simulink model "Q_2"  (R2019a)
settings: Solver=ode4  StartTime=0.0  StopTime=80  FixedStep=0.001  RelTol=1e-3  EnableMultiTasking=on
undefined symbols (not defined in the file or in its folder): attitude_control_1
settings Model: Creator=dell-  LastModifiedBy=lx
settings DataIOCC: LimitDataPoints=on  SaveFormat=Array  ReturnWorkspaceOutputs=off
settings OptimizationCC: LifeSpan=inf
settings DebuggingCC: SolverPrmCheckMsg=warning  SFUnexpectedBacktrackingDiag=warning  SFNoUnconditionalDefaultTransitionDiag=warning  SFExecutionAtInitializationDiag=none  ArithmeticOperatorsInVariantConditions=warning
settings HardwareCC: ProdBitPerPointer=32  ProdBitPerSizeT=32  ProdBitPerPtrDiffT=32  ProdLargestAtomicFloat=None  ProdIntDivRoundTo=Undefined  ProdEndianess=Unspecified  ProdWordSize=32  ProdHWDeviceType=32-bit Generic
settings ModelReferenceCC: PropagateSignalLabelsOutOfModel=off
settings SFSimCC: SimUseLocalCustomCode=off
settings RTWCC: RTWUseLocalCustomCode=off
settings CodeAppCC: StateflowObjectComments=on
settings GRTTargetCC: TargetLangStandard=C89/C90 (ANSI)  GeneratePreprocessorConditionals=Disable all
settings ConfigComp: CovMetricSettings=dw  CovHtmlReporting=on  CovSaveCumulativeToWorkspaceVar=on  CovSaveSingleToWorkspaceVar=on  CovExternalEMLEnable=off  CovSFcnEnable=off

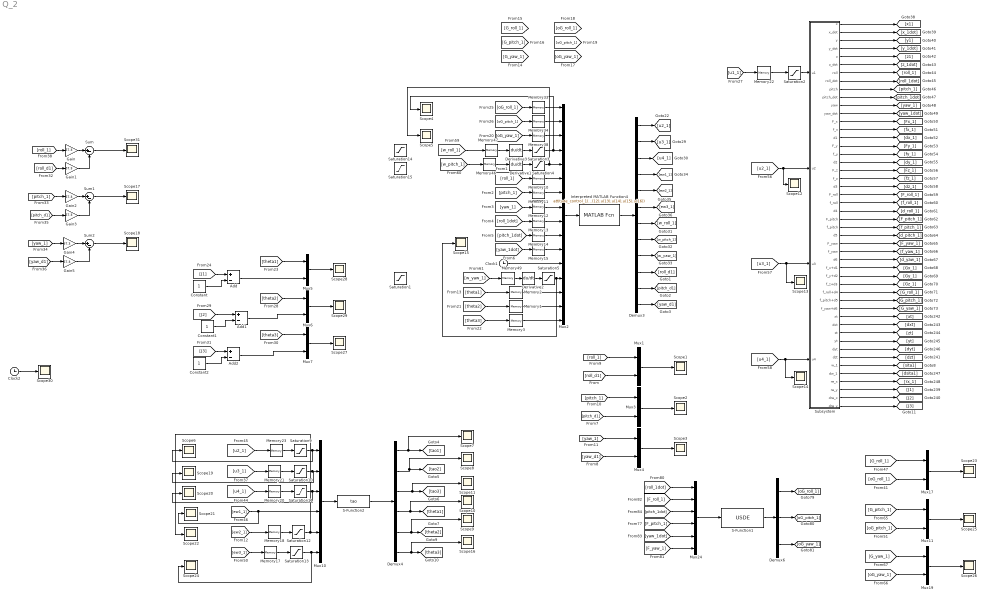
== system Q_2 ==
  Add : Sum  Inputs=+-
  Add1 : Sum  Inputs=+-
  Add2 : Sum  Inputs=+-
  Clock1 : Clock
  Clock2 : Clock
  Constant : Constant
  Constant1 : Constant
  Constant2 : Constant
  Demux3 : Demux  Outputs=12
  Demux4 : Demux  Outputs=6
  Demux6 : Demux  Outputs=3
  Derivative1 : Derivative
  Derivative2 : Derivative
  Derivative3 : Derivative
  Gain{,1..5} (6 alike) : Gain  Gain=57.3
  Interpreted MATLAB Function4 : MATLABFcn  MATLABFcn=attitude_control_1(u(1),u(2),u(3),u(4),u(5),u(6),u(7),u(8),u(9),u(10),u(11),u(12),u(13),u(14),u(15),u(16))  OutputDimensions=12  SampleTime=0.001
  Memory1 : Memory  InitialCondition=5.5
  Memory{10..11,13..15,18,20..23,33..34,38,46..47,49} (16 alike) : Memory
  Memory12 : Memory  InitialCondition=0.2
  Memory17 : Memory  InitialCondition=1
  Memory2 : Memory  InitialCondition=6
  Memory3 : Memory  InitialCondition=3
  Mux{1,3..7,11,17,19} (9 alike) : Mux  Inputs=2
  Mux10 : Mux  Inputs=6
  Mux2 : Mux  Inputs=16
  Mux24 : Mux  Inputs=6
  S-Function1 : S-Function  Priority=2  FunctionName=USDE  SFunctionDeploymentMode=off  EnableBusSupport=off
  S-Function2 : S-Function  FunctionName=tao  SFunctionDeploymentMode=off  EnableBusSupport=off
  Saturation1 : Saturate  UpperLimit=0.1  LowerLimit=-0.1
  Saturation10 : Saturate  UpperLimit=1.5  LowerLimit=-1
  Saturation11 : Saturate  UpperLimit=5  LowerLimit=-5
  Saturation12 : Saturate
  Saturation13 : Saturate  UpperLimit=0.2  LowerLimit=-0.2
  Saturation14 : Saturate  UpperLimit=0.2  LowerLimit=-0.2
  Saturation15 : Saturate
  Saturation2 : Saturate  UpperLimit=75  LowerLimit=-75
  Saturation3 : Saturate  UpperLimit=0.2  LowerLimit=-0.2
  Saturation4 : Saturate
  Saturation5 : Saturate  UpperLimit=0.1  LowerLimit=-0.1
  Saturation9 : Saturate  UpperLimit=1  LowerLimit=-1
  Scope{1..31} (31 alike) : Scope
  Subsystem : Subsystem  TreatAsAtomicUnit=on
      settings: RTWFcnNameOpts=Use subsystem name  RTWFileNameOpts=Use function name
  Sum : Sum  Inputs=|+-
  Sum1 : Sum  Inputs=|+-
  Sum2 : Sum  Inputs=|+-
  wires:
  [u1_1] -> Memory22/1
  [u2_1] -> Scope12/1, Subsystem/2(u2)
  [u3_1] -> Scope13/1, Subsystem/3(u3)
  [u4_1] -> Scope14/1, Subsystem/4(u4)
  Subsystem/1(x) -> [x1]
  Subsystem/2(x_dot) -> [x_1dot]
  Subsystem/3(y) -> [y1]
  Subsystem/4(y_dot) -> [y_1dot]
  Subsystem/5(z) -> [z1]
  Subsystem/6(z_dot) -> [z_1dot]
  Subsystem/7(roll) -> [roll_1]
  Subsystem/8(roll_dot) -> [roll_1dot]
  Subsystem/9(pitch) -> [pitch_1]
  Subsystem/10(pitch_dot) -> [pitch_1dot]
  Subsystem/11(yaw) -> [yaw_1]
  Subsystem/12(yaw_dot) -> [yaw_1dot]
  Subsystem/13(F_x) -> [Fx_1]
  Subsystem/14(f_x) -> [fx_1]
  Subsystem/15(d1) -> [dx_1]
  Subsystem/16(F_y) -> [Fy_1]
  Subsystem/17(f_y) -> [fy_1]
  Subsystem/18(d2) -> [dy_1]
  Subsystem/19(F_z) -> [Fz_1]
  Subsystem/20(f_z) -> [fz_1]
  Subsystem/21(d3) -> [dz_1]
  Subsystem/22(F_roll) -> [F_roll_1]
  Subsystem/23(f_roll) -> [f_roll_1]
  Subsystem/24(d4) -> [d_roll_1]
  Subsystem/25(F_pitch) -> [F_pitch_1]
  Subsystem/26(f_pitch) -> [f_pitch_1]
  Subsystem/27(d5) -> [d_pitch_1]
  Subsystem/28(F_yaw) -> [F_yaw_1]
  Subsystem/29(f_yaw) -> [f_yaw_1]
  Subsystem/30(d6) -> [d_yaw_1]
  Subsystem/36(f_yaw+d6) -> [G_yaw_1]
  Subsystem/35(f_pitch+d5) -> [G_pitch_1]
  Subsystem/34(f_roll+d4) -> [G_roll_1]
  Subsystem/33(f_z+d3) -> [Gz_1]
  Subsystem/32(f_y+d2) -> [Gy_1]
  Subsystem/31(f_x+d1) -> [Gx_1]
  Subsystem/41(dyt) -> [dyt]
  Subsystem/40(yt) -> [yt]
  Subsystem/39(zt) -> [zt]
  Subsystem/38(dxt) -> [dxt]
  Subsystem/42(dzt) -> [dzt]
  Subsystem/44(dw_1) -> [dsita1]
  Subsystem/45(re_x) -> [rx_1]
  Subsystem/46(re_y) -> [J1]
  Subsystem/47(dre_x) -> [J2]
  Subsystem/48(dre_y) -> [J3]
  Subsystem/37(xt) -> [xt]
  Interpreted MATLAB Function4/1 -> Demux3/1
  Mux2/1 -> Interpreted MATLAB Function4/1
  [oG_pitch_1] -> Memory34/1
  [oG_yaw_1] -> Memory38/1
  [oG_roll_1] -> Memory33/1
  Memory33/1 -> Mux2/1
  Memory34/1 -> Mux2/2
  Memory38/1 -> Mux2/3
  [roll_1] -> Memory10/1
  [yaw_1] -> Memory12/1
  [pitch_1] -> Memory11/1
  [roll_1dot] -> Memory13/1
  [pitch_1dot] -> Memory14/1
  [yaw_1dot] -> Memory15/1
  Demux3/4 -> [ew1_1]
  Demux3/5 -> [ew2_1]
  Demux3/6 -> [ew3_1]
  Demux3/1 -> [u2_1]
  Demux3/2 -> [u3_1]
  Demux3/3 -> [u4_1]
  [w_roll_1] -> Memory47/1
  [w_pitch_1] -> Memory46/1
  [w_yaw_1] -> Memory49/1
  Memory46/1 -> Derivative1/1
  Memory47/1 -> Derivative3/1
  Memory49/1 -> Derivative2/1
  Subsystem/43(w_1) -> [sita1]
  Memory22/1 -> Saturation2/1
  [oG_roll_1] -> Mux17/2
  Mux17/1 -> Scope23/1
  [oG_pitch_1] -> Mux11/2
  Mux11/1 -> Scope25/1
  [G_roll_1] -> Mux17/1
  [G_pitch_1] -> Mux11/1
  [oG_yaw_1] -> Mux19/2
  Mux19/1 -> Scope26/1
  [G_yaw_1] -> Mux19/1
  Mux24/1 -> S-Function1/1
  [roll_1dot] -> Mux24/1
  [F_roll_1] -> Mux24/2
  [pitch_1dot] -> Mux24/3
  [yaw_1dot] -> Mux24/5
  [F_pitch_1] -> Mux24/4
  [F_yaw_1] -> Mux24/6
  S-Function1/1 -> Demux6/1
  Demux6/3 -> [oG_yaw_1]
  Demux6/2 -> [oG_pitch_1]
  Demux6/1 -> [oG_roll_1]
  Saturation2/1 -> Subsystem/1(u1)
  Memory10/1 -> Mux2/6
  Memory11/1 -> Mux2/7
  Memory12/1 -> Mux2/8
  Memory13/1 -> Mux2/9
  Memory14/1 -> Mux2/10
  Memory15/1 -> Mux2/11
  Clock1/1 -> Mux2/12
  Demux3/7 -> [w_roll_1]
  Demux3/8 -> [w_pitch_1]
  Demux3/9 -> [w_yaw_1]
  Demux3/10 -> [roll_d1]
  Demux3/11 -> [pitch_d1]
  Demux3/12 -> [yaw_d1]
  [roll_1] -> Mux1/1
  Mux1/1 -> Scope1/1
  [roll_d1] -> Mux1/2
  Mux3/1 -> Scope2/1
  [pitch_1] -> Mux3/1
  [pitch_d1] -> Mux3/2
  Mux4/1 -> Scope3/1
  [yaw_1] -> Mux4/1
  [yaw_d1] -> Mux4/2
  [u4_1] -> Memory20/1
  [u3_1] -> Memory21/1
  Demux4/4 -> Scope10/1, [theta1]
  Demux4/6 -> Scope16/1, [theta3]
  [ew1_1] -> Mux10/4, Scope21/1
  Demux4/3 -> Scope11/1, [tao3]
  S-Function2/1 -> Demux4/1
  Demux4/1 -> Scope7/1, [tao1]
  Mux10/1 -> S-Function2/1
  Demux4/5 -> Scope9/1, [theta2]
  [ew3_1] -> Memory17/1
  [u2_1] -> Memory23/1
  Demux4/2 -> Scope8/1, [tao2]
  [ew2_1] -> Memory18/1
  [theta3] -> Memory3/1
  [theta1] -> Memory2/1
  [theta2] -> Memory1/1
  Memory2/1 -> Mux2/14
  Memory1/1 -> Mux2/15
  Memory3/1 -> Mux2/16
  [theta1] -> Mux5/1
  Mux7/1 -> Scope27/1
  Mux6/1 -> Scope29/1
  [J1] -> Add/1
  [theta3] -> Mux7/1
  [theta2] -> Mux6/1
  Mux5/1 -> Scope28/1
  Memory17/1 -> Saturation13/1
  Memory18/1 -> Saturation12/1
  Derivative2/1 -> Saturation5/1
  Derivative1/1 -> Saturation4/1
  Derivative3/1 -> Saturation3/1
  Memory20/1 -> Saturation11/1
  [roll_1] -> Gain/1
  [roll_d1] -> Gain1/1
  Sum/1 -> Scope31/1
  Sum1/1 -> Scope17/1
  [pitch_1] -> Gain2/1
  [pitch_d1] -> Gain3/1
  Sum2/1 -> Scope18/1
  [yaw_1] -> Gain4/1
  [yaw_d1] -> Gain5/1
  Memory23/1 -> Saturation9/1
  Memory21/1 -> Saturation10/1
  Saturation3/1 -> Scope4/1, Mux2/4
  Saturation4/1 -> Scope5/1, Mux2/5
  Saturation5/1 -> Scope15/1, Mux2/13
  Saturation9/1 -> Scope6/1, Mux10/1
  Saturation10/1 -> Scope19/1, Mux10/2
  Saturation11/1 -> Scope20/1, Mux10/3
  Saturation12/1 -> Scope22/1, Mux10/5
  Saturation13/1 -> Scope24/1, Mux10/6
  Gain/1 -> Sum/1
  Gain1/1 -> Sum/2
  Gain2/1 -> Sum1/1
  Gain3/1 -> Sum1/2
  Gain4/1 -> Sum2/1
  Gain5/1 -> Sum2/2
  Clock2/1 -> Scope30/1
  Add/1 -> Mux5/2
  Constant/1 -> Add/2
  [J2] -> Add1/1
  Constant1/1 -> Add1/2
  Add1/1 -> Mux6/2
  [J3] -> Add2/1
  Constant2/1 -> Add2/2
  Add2/1 -> Mux7/2

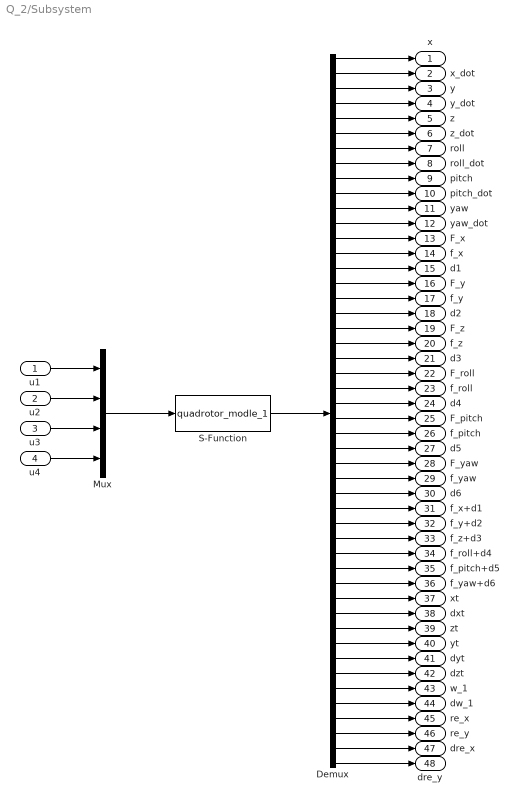
== system Q_2/Subsystem ==
  u1 : Inport
  u2 : Inport  Port=2
  u3 : Inport  Port=3
  u4 : Inport  Port=4
  Demux : Demux  Outputs=48
  Mux : Mux
  S-Function : S-Function  FunctionName=quadrotor_modle_1  SFunctionDeploymentMode=off  EnableBusSupport=off
  x : Outport
  x_dot : Outport  Port=2
  y : Outport  Port=3
  y_dot : Outport  Port=4
  z : Outport  Port=5
  z_dot : Outport  Port=6
  roll : Outport  Port=7
  roll_dot : Outport  Port=8
  pitch : Outport  Port=9
  pitch_dot : Outport  Port=10
  yaw : Outport  Port=11
  yaw_dot : Outport  Port=12
  F_x : Outport  Port=13
  f_x : Outport  Port=14
  d1 : Outport  Port=15
  F_y : Outport  Port=16
  f_y : Outport  Port=17
  d2 : Outport  Port=18
  F_z : Outport  Port=19
  f_z : Outport  Port=20
  d3 : Outport  Port=21
  F_roll : Outport  Port=22
  f_roll : Outport  Port=23
  d4 : Outport  Port=24
  F_pitch : Outport  Port=25
  f_pitch : Outport  Port=26
  d5 : Outport  Port=27
  F_yaw : Outport  Port=28
  f_yaw : Outport  Port=29
  d6 : Outport  Port=30
  f_x+d1 : Outport  Port=31
  f_y+d2 : Outport  Port=32
  f_z+d3 : Outport  Port=33
  f_roll+d4 : Outport  Port=34
  f_pitch+d5 : Outport  Port=35
  f_yaw+d6 : Outport  Port=36
  xt : Outport  Port=37
  dxt : Outport  Port=38
  zt : Outport  Port=39
  yt : Outport  Port=40
  dyt : Outport  Port=41
  dzt : Outport  Port=42
  w_1 : Outport  Port=43
  dw_1 : Outport  Port=44
  re_x : Outport  Port=45
  re_y : Outport  Port=46
  dre_x : Outport  Port=47
  dre_y : Outport  Port=48
  wires:
  u1/1 -> Mux/1
  u2/1 -> Mux/2
  u3/1 -> Mux/3
  u4/1 -> Mux/4
  Mux/1 -> S-Function/1
  S-Function/1 -> Demux/1
  Demux/1 -> x/1
  Demux/2 -> x_dot/1
  Demux/12 -> yaw_dot/1
  Demux/11 -> yaw/1
  Demux/10 -> pitch_dot/1
  Demux/9 -> pitch/1
  Demux/8 -> roll_dot/1
  Demux/7 -> roll/1
  Demux/6 -> z_dot/1
  Demux/5 -> z/1
  Demux/4 -> y_dot/1
  Demux/3 -> y/1
  Demux/13 -> F_x/1
  Demux/14 -> f_x/1
  Demux/15 -> d1/1
  Demux/16 -> F_y/1
  Demux/17 -> f_y/1
  Demux/18 -> d2/1
  Demux/19 -> F_z/1
  Demux/20 -> f_z/1
  Demux/21 -> d3/1
  Demux/22 -> F_roll/1
  Demux/23 -> f_roll/1
  Demux/24 -> d4/1
  Demux/25 -> F_pitch/1
  Demux/26 -> f_pitch/1
  Demux/27 -> d5/1
  Demux/28 -> F_yaw/1
  Demux/29 -> f_yaw/1
  Demux/30 -> d6/1
  Demux/31 -> f_x+d1/1
  Demux/32 -> f_y+d2/1
  Demux/33 -> f_z+d3/1
  Demux/36 -> f_yaw+d6/1
  Demux/35 -> f_pitch+d5/1
  Demux/34 -> f_roll+d4/1
  Demux/37 -> xt/1
  Demux/38 -> dxt/1
  Demux/39 -> zt/1
  Demux/40 -> yt/1
  Demux/41 -> dyt/1
  Demux/42 -> dzt/1
  Demux/43 -> w_1/1
  Demux/44 -> dw_1/1
  Demux/45 -> re_x/1
  Demux/46 -> re_y/1
  Demux/47 -> dre_x/1
  Demux/48 -> dre_y/1
